simulink library "dbs"  (Simulink 8.1)
settings: Solver=ode45  StartTime=0.0  StopTime=10.0  RelTol=1e-3
undefined symbols (not defined in the file or in its folder): AFCW_TargetVehicleTTCX_X_ms, AFCW_TargetVehRelSpeed_Y_kph, FALSE, KFCW_MaxDBSDeceleration_mps2, KFCW_MinDBSDeceleration_mps2, KFCW_WarnLightsDecel_mps2, KFCW_WarnLightSpeedThresh_mps, MFCW_DecelFromMap_mps2
libraries: hcu_lib x2
settings Model: Creator=xsellart  LastModifiedBy=tescamilla

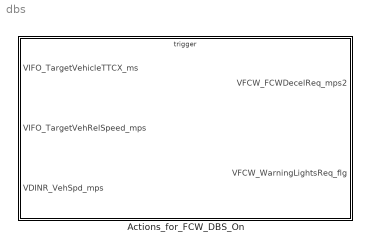
== system dbs ==
  Actions_for_FCW_DBS_On : Subsystem  TreatAsAtomicUnit=on

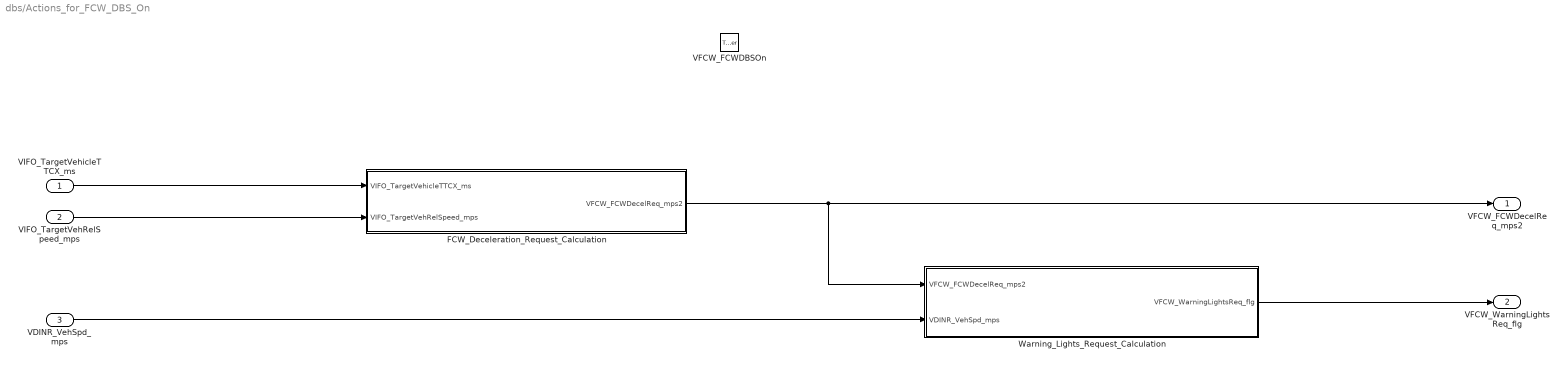
== system dbs/Actions_for_FCW_DBS_On ==
  VIFO_TargetVehicleTTCX_ms : Inport
  VIFO_TargetVehRelSpeed_mps : Inport  Port=2
  VDINR_VehSpd_mps : Inport  Port=3
  VFCW_FCWDBSOn : TriggerPort  TriggerType=function-call  StatesWhenEnabling=reset
      settings: AttributesFormatString=State = %<StatesWhenEnabling>
  FCW_Deceleration_Request_Calculation : Subsystem
  Warning_Lights_Request_Calculation : Subsystem
  VFCW_FCWDecelReq_mps2 : Outport  OutputWhenDisabled=reset  InitialOutput=0
  VFCW_WarningLightsReq_flg : Outport  Port=2  OutputWhenDisabled=reset  InitialOutput=FALSE
  wires:
  FCW_Deceleration_Request_Calculation/1(VFCW_FCWDecelReq_mps2) -> VFCW_FCWDecelReq_mps2/1, Warning_Lights_Request_Calculation/1(VFCW_FCWDecelReq_mps2)
  Warning_Lights_Request_Calculation/1(VFCW_WarningLightsReq_flg) -> VFCW_WarningLightsReq_flg/1
  VDINR_VehSpd_mps/1 -> Warning_Lights_Request_Calculation/2(VDINR_VehSpd_mps)
  VIFO_TargetVehRelSpeed_mps/1 -> FCW_Deceleration_Request_Calculation/2(VIFO_TargetVehRelSpeed_mps)
  VIFO_TargetVehicleTTCX_ms/1 -> FCW_Deceleration_Request_Calculation/1(VIFO_TargetVehicleTTCX_ms)

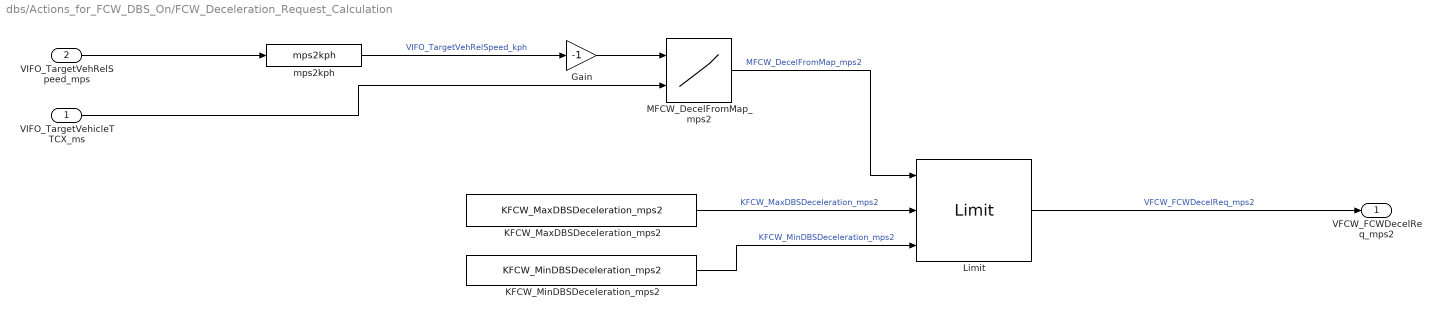
== system dbs/Actions_for_FCW_DBS_On/FCW_Deceleration_Request_Calculation ==
  VIFO_TargetVehicleTTCX_ms : Inport
  VIFO_TargetVehRelSpeed_mps : Inport  Port=2
  Gain : Gain  Gain=-1
  KFCW_MaxDBSDeceleration_mps2 : Constant  Value=KFCW_MaxDBSDeceleration_mps2
  KFCW_MinDBSDeceleration_mps2 : Constant  Value=KFCW_MinDBSDeceleration_mps2
  Limit : hcu_lib/Limit
  MFCW_DecelFromMap_mps2 : Lookup_n-D  BreakpointsForDimension1=AFCW_TargetVehRelSpeed_Y_kph  BreakpointsForDimension2=AFCW_TargetVehicleTTCX_X_ms  BreakpointsForDimension1Min=[0]  BreakpointsForDimension2Min=[0.7]  BreakpointsForDimension1Max=[200]  BreakpointsForDimension2Max=[5.6]  Table=MFCW_DecelFromMap_mps2  ExtrapMethod=Clip  UseLastTableValue=on  OutDataTypeStr=single  RndMeth=Simplest  InputSameDT=on
  mps2kph : hcu_lib/mps2kph
  VFCW_FCWDecelReq_mps2 : Outport  OutDataTypeStr=single
  wires:
  Limit/1 -> VFCW_FCWDecelReq_mps2/1  "VFCW_FCWDecelReq_mps2"
  MFCW_DecelFromMap_mps2/1 -> Limit/1  "MFCW_DecelFromMap_mps2"
  KFCW_MaxDBSDeceleration_mps2/1 -> Limit/2  "KFCW_MaxDBSDeceleration_mps2"
  KFCW_MinDBSDeceleration_mps2/1 -> Limit/3  "KFCW_MinDBSDeceleration_mps2"
  VIFO_TargetVehRelSpeed_mps/1 -> mps2kph/1
  mps2kph/1 -> Gain/1  "VIFO_TargetVehRelSpeed_kph"
  VIFO_TargetVehicleTTCX_ms/1 -> MFCW_DecelFromMap_mps2/2
  Gain/1 -> MFCW_DecelFromMap_mps2/1

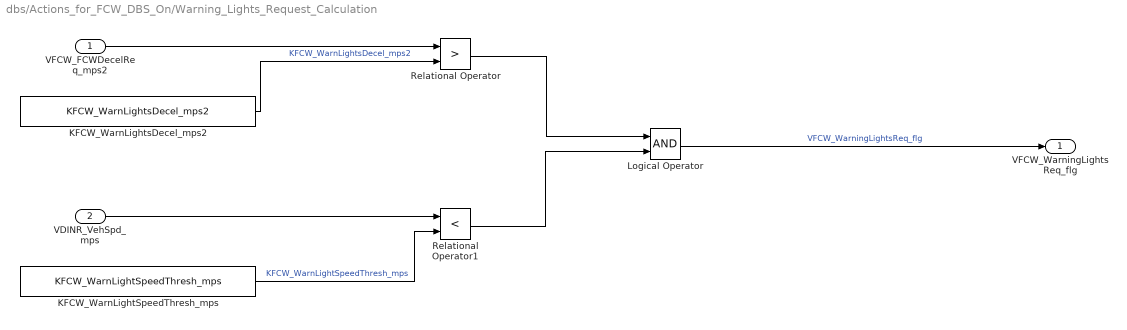
== system dbs/Actions_for_FCW_DBS_On/Warning_Lights_Request_Calculation ==
  VFCW_FCWDecelReq_mps2 : Inport
  VDINR_VehSpd_mps : Inport  Port=2
  KFCW_WarnLightSpeedThresh_mps : Constant  Value=KFCW_WarnLightSpeedThresh_mps
  KFCW_WarnLightsDecel_mps2 : Constant  Value=KFCW_WarnLightsDecel_mps2
  Logical Operator : Logic  AllPortsSameDT=off  OutDataTypeStr=boolean
  Relational Operator : RelationalOperator  Operator=>  OutDataTypeStr=boolean
  Relational Operator1 : RelationalOperator  Operator=<  OutDataTypeStr=boolean
  VFCW_WarningLightsReq_flg : Outport
  wires:
  KFCW_WarnLightsDecel_mps2/1 -> Relational Operator/2  "KFCW_WarnLightsDecel_mps2"
  VFCW_FCWDecelReq_mps2/1 -> Relational Operator/1
  KFCW_WarnLightSpeedThresh_mps/1 -> Relational Operator1/2  "KFCW_WarnLightSpeedThresh_mps"
  VDINR_VehSpd_mps/1 -> Relational Operator1/1
  Relational Operator/1 -> Logical Operator/1
  Relational Operator1/1 -> Logical Operator/2
  Logical Operator/1 -> VFCW_WarningLightsReq_flg/1  "VFCW_WarningLightsReq_flg"
